simulink model "snap_hdl_pfb_v3"  (R2021a)
settings: Solver=VariableStepDiscrete  StartTime=0.0  StopTime=16384  RelTol=1e-3
undefined symbols (not defined in the file): PFB, WB_PFB
libraries: xbsIndex_r4 x451, simulink x4, xps_library x2, casper_library_misc x2
(part 1 of 6)
settings Model: Creator=wei  LastModifiedBy=wei
settings SolverCC: AlgebraicLoopSolver=TrustRegion
settings OptimizationCC: DefaultParameterBehavior=Inlined
settings DebuggingCC: SFMachineParentedDataDiag=warning
settings SFSimCC: CustomCodeUndefinedFunction=UseInterfaceOnly

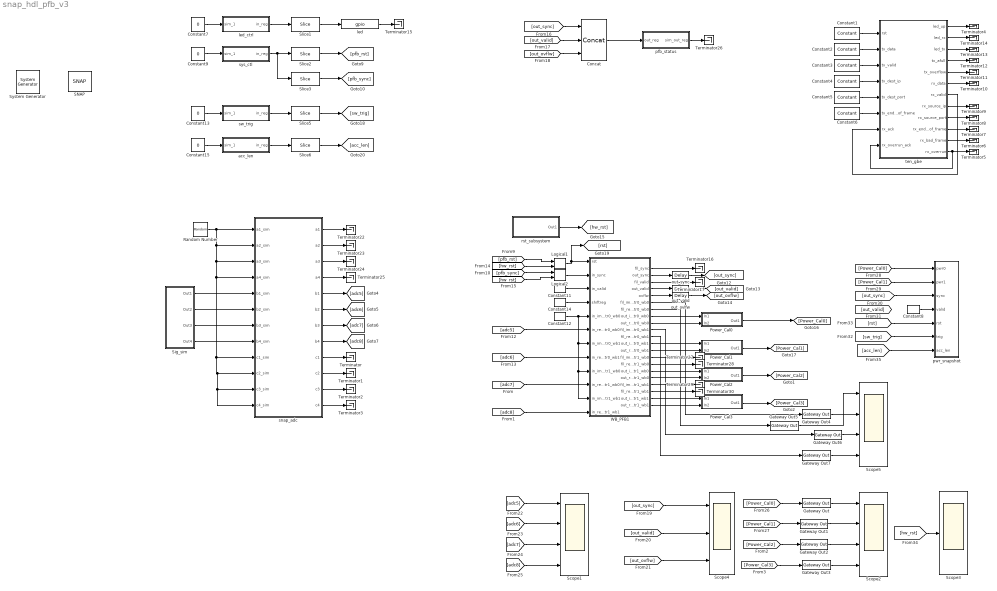
== system snap_hdl_pfb_v3 ==
  " System Generator" : xbsIndex_r4/ System Generator  Tag=genX  xilinxfamily=kintex7  part=xc7k160t  speed=-2  package=ffg676  synthesis_tool=XST  clock_wrapper=Clock Enables  directory=/data/Wei/casper_hdl/snap_hdl_tut/snap_hdl_pfb_v2/sysgen  proj_type=Vivado  Synth_file=Vivado Synthesis Defaults  Impl_file=Vivado Implementation Defaults  testbench=off  simulink_period=1  sysclk_period=4  dcm_input_clock_period=10  incr_netlist=off  trim_vbits=Everywhere in SubSystem  dbl_ovrd=According to Block Masks  core_generation=According to Block Masks  run_coregen=off  deprecated_control=off  eval_field=0  block_type=sysgen
  Concat : xbsIndex_r4/Concat  num_inputs=3  dbl_ovrd=off  block_type=concat
  Constant1 : xbsIndex_r4/Constant  const=0  gui_display_data_type=Boolean  arith_type=Boolean  n_bits=16  bin_pt=14  preci_type=Single  exp_width=8  frac_width=24  explicit_period=on  period=1  equ=P=C  opselect=C  inp2=PCIN>>17  opr=+  inp1=P  carry=CIN  dbl_ovrd=off  block_type=constant
  Constant11 : xbsIndex_r4/Constant  const=1.0  gui_display_data_type=Fixed-point  arith_type=Unsigned  n_bits=1  bin_pt=0  preci_type=Single  exp_width=8  frac_width=24  explicit_period=on  period=1  equ=P=C  opselect=C  inp2=PCIN>>17  opr=+  inp1=P  carry=CIN  dbl_ovrd=off  block_type=constant
  Constant12 : xbsIndex_r4/Constant  const=0  gui_display_data_type=Fixed-point  arith_type=Unsigned  n_bits=8  bin_pt=0  preci_type=Single  exp_width=8  frac_width=24  explicit_period=on  period=1  equ=P=C  opselect=C  inp2=PCIN>>17  opr=+  inp1=P  carry=CIN  dbl_ovrd=off  block_type=constant
  Constant{7,9,13,15} (4 alike) : Constant  Value=0  SampleTime=-1
  Constant14 : xbsIndex_r4/Constant  const=1023  gui_display_data_type=Fixed-point  arith_type=Unsigned  n_bits=10  bin_pt=0  preci_type=Single  exp_width=8  frac_width=24  explicit_period=on  period=1  equ=P=C  opselect=C  inp2=PCIN>>17  opr=+  inp1=P  carry=CIN  dbl_ovrd=off  block_type=constant
  Constant2 : xbsIndex_r4/Constant  const=0  gui_display_data_type=Fixed-point  arith_type=Unsigned  n_bits=64  bin_pt=0  preci_type=Single  exp_width=8  frac_width=24  explicit_period=on  period=1  equ=P=C  opselect=C  inp2=PCIN>>17  opr=+  inp1=P  carry=CIN  dbl_ovrd=off  block_type=constant
  Constant3 : xbsIndex_r4/Constant  const=0  gui_display_data_type=Boolean  arith_type=Boolean  n_bits=16  bin_pt=14  preci_type=Single  exp_width=8  frac_width=24  explicit_period=on  period=1  equ=P=C  opselect=C  inp2=PCIN>>17  opr=+  inp1=P  carry=CIN  dbl_ovrd=off  block_type=constant
  Constant4 : xbsIndex_r4/Constant  const=0  gui_display_data_type=Fixed-point  arith_type=Unsigned  n_bits=32  bin_pt=0  preci_type=Single  exp_width=8  frac_width=24  explicit_period=on  period=1  equ=P=C  opselect=C  inp2=PCIN>>17  opr=+  inp1=P  carry=CIN  dbl_ovrd=off  block_type=constant
  Constant5 : xbsIndex_r4/Constant  const=0  gui_display_data_type=Fixed-point  arith_type=Unsigned  n_bits=16  bin_pt=0  preci_type=Single  exp_width=8  frac_width=24  explicit_period=on  period=1  equ=P=C  opselect=C  inp2=PCIN>>17  opr=+  inp1=P  carry=CIN  dbl_ovrd=off  block_type=constant
  Constant6 : xbsIndex_r4/Constant  const=0  gui_display_data_type=Boolean  arith_type=Boolean  n_bits=32  bin_pt=0  preci_type=Single  exp_width=8  frac_width=24  explicit_period=on  period=1  equ=P=C  opselect=C  inp2=PCIN>>17  opr=+  inp1=P  carry=CIN  dbl_ovrd=off  block_type=constant
  Constant8 : xbsIndex_r4/Constant  const=1.0  gui_display_data_type=Fixed-point  arith_type=Unsigned  n_bits=1  bin_pt=0  preci_type=Single  exp_width=8  frac_width=24  explicit_period=on  period=1  equ=P=C  opselect=C  inp2=PCIN>>17  opr=+  inp1=P  carry=CIN  dbl_ovrd=off  block_type=constant
  Gateway Out{,1..7} (8 alike) : xbsIndex_r4/Gateway Out  inherit_from_input=off  hdl_port=on  rows=1  columns=1  UseAsDAC=off  DACChannel='1'  interface=None  automatic_assignment=on  address_offset=hex2dec('00')  intf_name=''  intf_description=''  timing_constraint=None  locs_specified=off  LOCs={}  io_standard={}  block_type=gatewayout
  Logical1 : xbsIndex_r4/Logical  logical_function=OR  inputs=2  en=off  latency=0  precision=Full  arith_type=Unsigned  n_bits=8  bin_pt=2  align_bp=on  dbl_ovrd=off  block_type=logical
      settings: xl_area=[0, 0, 0, 0, 0, 0, 0]
  Logical2 : xbsIndex_r4/Logical  logical_function=OR  inputs=2  en=off  latency=0  precision=Full  arith_type=Unsigned  n_bits=8  bin_pt=2  align_bp=on  dbl_ovrd=off  block_type=logical
      settings: xl_area=[0, 0, 0, 0, 0, 0, 0]
  Power_Cal0 : Subsystem
  Power_Cal1 : Subsystem
  Power_Cal2 : Subsystem
  Power_Cal3 : Subsystem
  Random Number : RandomNumber  SampleTime=0.1
  SNAP : xps_library/Platforms/SNAP  Tag=xps:xsg  hw_sys=SNAP:xc7k160t  clk_src=adc0_clk  clk_rate=250  use_microblaze=on  sample_period=1  synthesis_tool=XST
      settings: SourceProductName=CASPER XPS Blockset
  Scope1 : Scope  NumInputPorts=4
  Scope2 : Scope  NumInputPorts=4
  Scope3 : Scope
  Scope4 : Scope  NumInputPorts=3
  Scope5 : Scope  NumInputPorts=4
  Sig_sim : Subsystem
  Slice1 : xbsIndex_r4/Slice  nbits=1  boolean_output=on  mode=Lower Bit Location + Width  bit1=0  base1=MSB of Input  bit0=0  base0=LSB of Input  dbl_ovrd=off  block_type=slice
  Slice2 : xbsIndex_r4/Slice  nbits=1  boolean_output=on  mode=Lower Bit Location + Width  bit1=0  base1=MSB of Input  bit0=0  base0=LSB of Input  dbl_ovrd=off  block_type=slice
  Slice3 : xbsIndex_r4/Slice  nbits=1  boolean_output=on  mode=Lower Bit Location + Width  bit1=0  base1=MSB of Input  bit0=1  base0=LSB of Input  dbl_ovrd=off  block_type=slice
  Slice5 : xbsIndex_r4/Slice  nbits=10  boolean_output=on  mode=Lower Bit Location + Width  bit1=0  base1=MSB of Input  bit0=0  base0=LSB of Input  dbl_ovrd=off  block_type=slice
  Slice6 : xbsIndex_r4/Slice  nbits=24  boolean_output=off  mode=Lower Bit Location + Width  bit1=0  base1=MSB of Input  bit0=0  base0=LSB of Input  dbl_ovrd=off  block_type=slice
  Terminator{,1..17,22..30} (27 alike) : Terminator
  WB_PFB1 : Subsystem  AncestorBlock=PFB/WB_PFB  mask(Wideband Polyphase Filterbank Block){use_separate=off, use_fft_shift=off, use_reorder=on, alt_output=off, wb_factor=2, nof_points=10, nof_taps=4, nof_wb_streams=2, nof_chan=0, xtra_dat_sigs=off, big_endian_wb_in=off, use_prefilter=on, dont_flip_channels=on, out_gain_w=0, win="hanning", fwidth=1.0, backoff_w=0, fil_in_dat_w=8, fil_out_dat_w=14, fil_coef_dat_w=10, twid_dat_w=18, fft_stage_dat_w=20, fft_out_dat_w=20, fft_guard_enable=off, fft_guard_w=2, fft_ovflw_behav="WRAP", fft_use_round=1, pipe_reo_in_place=off, use_dsp="YES", use_variant="4DSP", fft_ram_primitive="block", max_addr_w=8, fil_ram_primitive="block", vendor_technology=Xilinx}
      mask prompts: use_separate "Separate re/im outputs"; use_fft_shift "Reorder frequencies"; use_reorder "Bit reverse output"; alt_output "Alter output data stream"; wb_factor "Wideband factor"; nof_points "Number of points (2^nof_pts)"; nof_taps "Number of taps"; nof_wb_streams "Number of wideband streams"; nof_chan "Number of channels (2^nof_chan)"; xtra_dat_sigs "Extra control signals"; big_endian_wb_in "Big endian input data"; use_prefilter "Enable prefilter"; dont_flip_channels "Don't flip channels"; out_gain_w "Output gain width"; win "Window function"; backoff_w "Filter backoff width"; fil_in_dat_w "Prefilter input data width"; fil_out_dat_w "Prefilter output data width"; fil_coef_dat_w "Prefilter coefficient data width"; twid_dat_w "FFT twiddle data width"; fft_stage_dat_w "FFT stage data width"; fft_out_dat_w "FFT output data width"; fft_guard_enable "Guard FFT input data"; fft_guard_w "FFT guard data width"; fft_ovflw_behav "FFT overflow behaviour"; fft_use_round "FFT rounding mode: 0-Truncate, 1-Round Even, 2-Round Infinite"; pipe_reo_in_place "Use single pipelined FFT reorder buffer"; use_dsp "Use DSP for Cmults"; use_variant "Cmult options"; fft_ram_primitive "FFT Ram Primitive"; max_addr_w "Twiddle Max Address Width"; fil_ram_primitive "Prefilter Ram Primitive"; vendor_technology "Vendor technology"
      mask help: The Wideband Poly Phase FilterBank can process a datastream that is partly applied in serial and partly applied in parallel. It consists of a Poly Phase Filter (PPF) and a Fast Fourier Transform (FFT). It distinguishes from a single FFT by the PPF, that acts as a window function to produce a flat response across the channel, and excellent suppression of out-of-band signals.
      mask init:
      | Simulink.Block.eval([gcb, '/wb_pfb']);
      |  
      | wb_pfb_subsys2bb_knit();
      mask Help: https://casper-dspdevel.readthedocs.io/en/latest/wideband_pfb.html
      mask Callback use_separate:
      | enab = get_param(gcb,'use_separate');
      | 
      | % Set the 'MaskVisibilities' property for each parameters
      | if strcmp(enab,'on')
      |     set_param(gcb,'use_reorder','on');
      |     set_param(gcb,'use_fft_shift','off');
      |     set_param(gcb,'MaskEnables',{'on','off','off','on','on','on','on','on','on','on','on','on','on','on','on','on','on','on','on','on','on','on','on','on','on','on','on','on','on','on','on','on','on','on'});
      | else
      |     set_param(gcb,'MaskEnables',{'on','on','on','on','on','on','on','on','on','on','on','on','on','on','on','on','on','on','on','on','on','on','on','on','on','on','on','on','on','on','on','on','on','on'});
      | end
      mask Callback use_fft_shift:
      | enab = get_param(gcb,'use_fft_shift');
      | 
      | % Set the 'MaskVisibilities' property for each parameters
      | if strcmp(enab,'on')
      |     set_param(gcb,'use_reorder','on');
      |     set_param(gcb,'MaskEnables',{'on','on','off','on','on','on','on','on','on','on','on','on','on','on','on','on','on','on','on','on','on','on','on','on','on','on','on','on','on','on','on','on','on','on'});
      | else
      |     set_param(gcb,'MaskEnables',{'on','on','on','on','on','on','on','on','on','on','on','on','on','on','on','on','on','on','on','on','on','on','on','on','on','on','on','on','on','on','on','on','on','on'});
      | end
      mask TypeOptions win: "hanning" | "hamming" | "blackman"
      mask Callback fft_guard_enable:
      | enab = get_param(gcb,'fft_guard_enable');
      | 
      | % Set the 'MaskVisibilities' property for each parameters
      | if strcmp(enab,'on')
      |     set_param(gcb,'MaskVisibilities',{'on','on','on','on','on','on','on','on','on','on','on','on','on','on','on','on','on','on','on','on','on','on','on','on','on','on','on','on','on','on','on','on','on','on'});
      | else
      |     set_param(gcb,'MaskVisibilities',{'on','on','on','on','on','on','on','on','on','on','on','on','on','on','on','on','on','on','on','on','on','on','on','on','off','on','on','on','on','on','on','on','on','on'});
      | end
      mask TypeOptions fft_ovflw_behav: "SATURATE" | "WRAP"
      mask TypeOptions fft_use_round: 0 | 1 | 2
      mask TypeOptions use_dsp: "YES" | "NO"
      mask TypeOptions use_variant: "4DSP" | "3DSP"
      mask TypeOptions fft_ram_primitive: "block" | "distributed" | "ultra" | "auto"
      mask TypeOptions fil_ram_primitive: "block" | "distributed" | "ultra" | "auto"
      mask TypeOptions vendor_technology: Xilinx | UniBoard
      mask DialogControl DescTextVar Prompt: The wpfb unit is a Wideband Poly Phase FilterBank which can process a datastream that is partly applied in serial and partly applied in parallel. It consists of a Poly Phase Filter (PPF) and a Fast Fourier Transform (FFT). The wpfb distinguishes from a single FFT by the PPF that functions as a window function in order to produce a flat response across the channel, but also provides excellent suppression of out-of-band signals. https://casper-dspdevel.readthedocs.io/en/latest/wideband_pfb.html
      mask DialogControl pfb_params Prompt: PFB Parameters
      mask DialogControl pfb Prompt: PFB
      mask DialogControl filter Prompt: FILTER
      mask DialogControl fft Prompt: FFT
      mask DialogControl synth Prompt: SYNTH/IMP
  acc_len : Subsystem  Tag=xps:sw_reg  AncestorBlock=xps_library/Memory/software_register  mask(swreg){io_dir=From Processor, io_delay=0, init_val=0, sample_period=1, names=reg, bitwidths=32, bin_pts=0, arith_types=0, sim_port=on, show_format=on}
      mask prompts: io_dir "I/O direction"; io_delay "I/O delay"; init_val "Initial Value"; sample_period "Sample period"; names "Bitfield names [msb...lsb]"; bitwidths "Bitfield widths"; bin_pts "Bitfield binary pts"; arith_types "Bitfield types, ufix=0, fix=1, bool=2"; sim_port "Provide sim input/output?"; show_format "Print format string?"
      mask help: A 32-bit software-accessible register. Can be divided into bitfields of varying widths and types using the fields in the block mask.
      mask init:
      | swreg_init(gcb)
      settings: AttributesFormatString=1input:uf32.0 = 32 bits
      mask TypeOptions io_dir: To Processor | From Processor
      mask Callback io_dir:
      | mask_enables = get_param(gcb, 'MaskEnables');
      | mask_names = get_param(gcb, 'MaskNames');
      | if strcmp(get_param(gcb, 'io_dir'), 'To Processor'),
      |     mask_enables{ismember(mask_names, 'sample_period')} = 'off';
      | else
      |     mask_enables{ismember(mask_names, 'sample_period')} = 'on';
      | end
      | set_param(gcb, 'MaskEnables', mask_enables);
      mask DialogControl ParameterTabVar0 Prompt: Setup
  led : xps_library/IO/gpio  Tag=xps:gpio  io_group_params_forwarded=on  io_group=ROACH:led  io_group_real=led  io_group_custom=0  io_dir=out  arith_type=Boolean  bitwidth=1  bin_pt=0  bit_index=0  sample_period=1  use_single_ended=off  use_ddr=off  reg_iob=on  reg_clk_phase=0  termination=None  use_iodelay=off
      settings: SourceProductName=CASPER XPS Blockset
  led_ctrl : Subsystem  Tag=xps:sw_reg  AncestorBlock=xps_library/Memory/software_register  mask(swreg){io_dir=From Processor, io_delay=0, init_val=0, sample_period=1, names=reg, bitwidths=32, bin_pts=0, arith_types=0, sim_port=on, show_format=on}
      mask prompts: io_dir "I/O direction"; io_delay "I/O delay"; init_val "Initial Value"; sample_period "Sample period"; names "Bitfield names [msb...lsb]"; bitwidths "Bitfield widths"; bin_pts "Bitfield binary pts"; arith_types "Bitfield types, ufix=0, fix=1, bool=2"; sim_port "Provide sim input/output?"; show_format "Print format string?"
      mask help: A 32-bit software-accessible register. Can be divided into bitfields of varying widths and types using the fields in the block mask.
      mask init:
      | swreg_init(gcb)
      settings: AttributesFormatString=1input:uf32.0 = 32 bits
      mask TypeOptions io_dir: To Processor | From Processor
      mask Callback io_dir:
      | mask_enables = get_param(gcb, 'MaskEnables');
      | mask_names = get_param(gcb, 'MaskNames');
      | if strcmp(get_param(gcb, 'io_dir'), 'To Processor'),
      |     mask_enables{ismember(mask_names, 'sample_period')} = 'off';
      | else
      |     mask_enables{ismember(mask_names, 'sample_period')} = 'on';
      | end
      | set_param(gcb, 'MaskEnables', mask_enables);
      mask DialogControl ParameterTabVar0 Prompt: Setup
  out_ovlfw : xbsIndex_r4/Delay  rst=off  infoeditControl=Selection of Reset will increase slice count due to use of real FFs and instead of SRLs  en=off  latency=5  reg_retiming=off  dbl_ovrd=off  block_type=delay
  out_sync : xbsIndex_r4/Delay  rst=off  infoeditControl=Selection of Reset will increase slice count due to use of real FFs and instead of SRLs  en=off  latency=5  reg_retiming=off  dbl_ovrd=off  block_type=delay
  out_valid : xbsIndex_r4/Delay  rst=off  infoeditControl=Selection of Reset will increase slice count due to use of real FFs and instead of SRLs  en=off  latency=5  reg_retiming=off  dbl_ovrd=off  block_type=delay
  pfb_status : Subsystem  Tag=xps:sw_reg  AncestorBlock=xps_library/Memory/software_register  mask(swreg){io_dir=To Processor, io_delay=0, init_val=0, sample_period=1, names=reg, bitwidths=12, bin_pts=0, arith_types=0, sim_port=on, show_format=off}
      mask prompts: io_dir "I/O direction"; io_delay "I/O delay"; init_val "Initial Value"; sample_period "Sample period"; names "Bitfield names [msb...lsb]"; bitwidths "Bitfield widths"; bin_pts "Bitfield binary pts"; arith_types "Bitfield types, ufix=0, fix=1, bool=2"; sim_port "Provide sim input/output?"; show_format "Print format string?"
      mask help: A 32-bit software-accessible register. Can be divided into bitfields of varying widths and types using the fields in the block mask.
      mask init:
      | swreg_init(gcb)
      settings: AttributesFormatString=1output
      mask TypeOptions io_dir: To Processor | From Processor
      mask Callback io_dir:
      | mask_enables = get_param(gcb, 'MaskEnables');
      | mask_names = get_param(gcb, 'MaskNames');
      | if strcmp(get_param(gcb, 'io_dir'), 'To Processor'),
      |     mask_enables{ismember(mask_names, 'sample_period')} = 'off';
      | else
      |     mask_enables{ismember(mask_names, 'sample_period')} = 'on';
      | end
      | set_param(gcb, 'MaskEnables', mask_enables);
      mask DialogControl ParameterTabVar0 Prompt: Setup
  pwr_snapshot : Subsystem
  rst_subsystem : Subsystem
  snap_adc : Subsystem  Tag=xps:snap_adc  AncestorBlock=xps_library/ADCs/snap_adc  mask(adc_snap){sample_rate=500, snap_inputs=6, adc_resolution=8}
      mask prompts: sample_rate "Sample rate (MHz)"; snap_inputs "Number of inputs per snap"; adc_resolution "Resolution of ADC (number of bit)"
      mask help: Interface to the 3 adc chips on the SNAP board. Please see Help for instructions on parameter settings
      mask init:
      | adc_snap_init(gcb);
      mask Help:
      | This is the CASPER "yellow block" for the ADCs on the SNAP board.
      | Each ADC chip accepts four inputs.
      | 
      | Maximum sample rate f (Mega samples per second)
      | 
      | Number of inputs         3                6                12
      | Resolution 8 bits          f=1000      f=500         f=250
      | Resolution 12 bits        f=640        f=320         f=160
      | 
      | Resolution 12 bits is available when SNAP board is upgraded with HMCAD1520 ADC chips
      mask TypeOptions snap_inputs: 3 | 6 | 12
      mask TypeOptions adc_resolution: 8 | 12
  sw_trig : Subsystem  Tag=xps:sw_reg  AncestorBlock=xps_library/Memory/software_register  mask(swreg){io_dir=From Processor, io_delay=0, init_val=0, sample_period=1, names=reg, bitwidths=32, bin_pts=0, arith_types=0, sim_port=on, show_format=on}
      mask prompts: io_dir "I/O direction"; io_delay "I/O delay"; init_val "Initial Value"; sample_period "Sample period"; names "Bitfield names [msb...lsb]"; bitwidths "Bitfield widths"; bin_pts "Bitfield binary pts"; arith_types "Bitfield types, ufix=0, fix=1, bool=2"; sim_port "Provide sim input/output?"; show_format "Print format string?"
      mask help: A 32-bit software-accessible register. Can be divided into bitfields of varying widths and types using the fields in the block mask.
      mask init:
      | swreg_init(gcb)
      settings: AttributesFormatString=1input:uf32.0 = 32 bits
      mask TypeOptions io_dir: To Processor | From Processor
      mask Callback io_dir:
      | mask_enables = get_param(gcb, 'MaskEnables');
      | mask_names = get_param(gcb, 'MaskNames');
      | if strcmp(get_param(gcb, 'io_dir'), 'To Processor'),
      |     mask_enables{ismember(mask_names, 'sample_period')} = 'off';
      | else
      |     mask_enables{ismember(mask_names, 'sample_period')} = 'on';
      | end
      | set_param(gcb, 'MaskEnables', mask_enables);
      mask DialogControl ParameterTabVar0 Prompt: Setup
  sys_ctl : Subsystem  Tag=xps:sw_reg  AncestorBlock=xps_library/Memory/software_register  mask(swreg){io_dir=From Processor, io_delay=0, init_val=0, sample_period=1, names=reg, bitwidths=32, bin_pts=0, arith_types=0, sim_port=on, show_format=on}
      mask prompts: io_dir "I/O direction"; io_delay "I/O delay"; init_val "Initial Value"; sample_period "Sample period"; names "Bitfield names [msb...lsb]"; bitwidths "Bitfield widths"; bin_pts "Bitfield binary pts"; arith_types "Bitfield types, ufix=0, fix=1, bool=2"; sim_port "Provide sim input/output?"; show_format "Print format string?"
      mask help: A 32-bit software-accessible register. Can be divided into bitfields of varying widths and types using the fields in the block mask.
      mask init:
      | swreg_init(gcb)
      settings: AttributesFormatString=1input:uf32.0 = 32 bits
      mask TypeOptions io_dir: To Processor | From Processor
      mask Callback io_dir:
      | mask_enables = get_param(gcb, 'MaskEnables');
      | mask_names = get_param(gcb, 'MaskNames');
      | if strcmp(get_param(gcb, 'io_dir'), 'To Processor'),
      |     mask_enables{ismember(mask_names, 'sample_period')} = 'off';
      | else
      |     mask_enables{ismember(mask_names, 'sample_period')} = 'on';
      | end
      | set_param(gcb, 'MaskEnables', mask_enables);
      mask DialogControl ParameterTabVar0 Prompt: Setup
  ten_gbe : Subsystem  Tag=xps:ten_gbe  AncestorBlock=xps_library/IO/ten_gbe  mask(ten_gbe){flavour=sfp+, slot=0, port_r1=1, port_r2_cx4=0, port_r2_sfpp=0, rx_dist_ram=off, large_frames=on, show_param=on, pre_emph_r2=1.07, pre_emph=3, post_emph_r2=0.18, rxeqmix_r2=7, swing_r2=940, swing=800, fab_en=off, fab_mac=hex2dec('123456780000'), fab_ip=192*(2^24) + 168*(2^16) + 5*(2^8) + 20*(2^0), fab_udp=10000, fab_gate=1, cpu_rx_en=on, cpu_tx_en=on, ttl=hex2dec('FF'), promisc_mode=off, debug_ctr_width=16, txctr=off, txerrctr=off, txerrctr_len=100, txofctr=off, txfullctr=off, txvldctr=off, txsnaplen=0 - no snap, rxctr=off, rxerrctr=off, rxerrctr_len=100, rxofctr=off, rxbadctr=off, rxvldctr=off, rxeofctr=off, rxsnaplen=0 - no snap}
      mask prompts: flavour "Mezzanine card flavour"; slot "Card slot"; port_r1 "Port"; port_r2_cx4 "Port"; port_r2_sfpp "Port"; rx_dist_ram "Shallow RX Fifo (Beware overruns!)"; large_frames "Enable Large TX Frames (8k+512)"; show_param "---------------------- Show Implementation Parameters -----------------------------------------------------------------------------------"; pre_emph_r2 "Pre-emphasis (dB)"; pre_emph "Pre-emphasis"; post_emph_r2 "Post-emphasis (dB)"; rxeqmix_r2 "Receive equalisation"; swing_r2 "Driver Swing Control (mVppd)"; swing "Differential swing"; fab_en "Enable fabric on startup"; fab_mac "Fabric MAC Address"; fab_ip "Fabric IP Address"; fab_udp "Fabric UDP Port"; fab_gate "Fabric Gateway"; cpu_rx_en "Enable CPU RX"; cpu_tx_en "Enable CPU TX"; promisc_mode "Promiscuous mode"; debug_ctr_width "Debug counter width"; txctr "TX - core_txctr"; txerrctr "TX packet length error - core_txerrctr"; txerrctr_len "-- expected TX packet length"; txofctr "TX overflow - core_txofctr"; txfullctr "TX full - core_txfullctr"; txvldctr "TX valid cycle - core_txvldctr"; txsnaplen "TX snapshot length"; rxctr "RX - core_rxctr"; rxerrctr "RX packet length error - core_rxerrctr"; rxerrctr_len "-- expected RX packet length"; rxofctr "RX overflow - core_rxofctr"; rxbadctr "RX bad - core_rxbadctr"; rxvldctr "RX valid cycle - core_rxvldctr"; rxeofctr "RX eof - core_rxeofctr"; rxsnaplen "RX snapshot length"
      mask help: This block sends and receives UDP frames (packets). It accepts a 64 bit wide data stream with user-determined frame breaks. The data stream is wrapped in a UDP frame for transmission. Incoming UDP packets are unwrapped and the data presented as a 64 bit wide stream.
      mask init:
      | temp = eval(get_param(gcb, 'debug_ctr_width'));
      | if temp <= 0,
      |     error('Debug counters cannot be ltoet zero.');
      | end
      | tengbe_mask(gcb)
      mask TypeOptions flavour: sfp+ | cx4
      mask Callback flavour: tengbe_callback
      mask TypeOptions slot: 0 | 1
      mask TypeOptions port_r1: 0 | 1 | 2 | 3
      mask TypeOptions port_r2_cx4: 0 | 1 | 2
      mask TypeOptions port_r2_sfpp: 0 | 1 | 2 | 3
      mask Callback show_param: tengbe_callback
      mask TypeOptions pre_emph_r2: 0.15 | 0.3 | 0.45 | 0.61 | 0.74 | 0.91 | 1.07 | 1.25 | 1.36 | 1.55 | 1.74 | 1.94 | 2.11 | 2.32 | 2.54 | 2.77
      mask TypeOptions pre_emph: 0 | 1 | 2 | 3
      mask TypeOptions post_emph_r2: 0.18 | 0.19 | 0.2 | 0.39 | 0.63 | 0.82 | 1.07 | 1.32 | 1.6 | 1.65 | 1.94 | 2.21 | 2.52 | 2.76 | 3.08 | 3.41 | 3.77 | 3.97 | 4.36 | 4.73 | 5.16 | 5.47 | 5.93 | 6.38 | 6.89
      mask TypeOptions rxeqmix_r2: 0 | 1 | 2 | 3 | 4 | 5 | 6 | 7
      mask TypeOptions swing_r2: 110 | 210 | 310 | 400 | 480 | 570 | 660 | 740 | 810 | 880 | 940 | 990 | 1040 | 1080 | 1110 | 1130
      mask TypeOptions swing: 400 | 500 | 600 | 700 | 800
      mask Callback txerrctr:
      | blk = gcb;
      | mask_visibilities = get_param(blk, 'MaskVisibilities');
      | mask_names = get_param(blk, 'MaskNames');
      | if strcmp(get_param(blk, 'txerrctr'), 'on')
      |     mask_visibilities{ismember(mask_names, 'txerrctr_len')} = 'on';
      | else
      |     mask_visibilities{ismember(mask_names, 'txerrctr_len')} = 'off';
      | end
      | set_param(blk, 'MaskVisibilities', mask_visibilities);
      mask TypeOptions txsnaplen: 0 - no snap | 256 | 512 | 1024 | 2048 | 4096 | 8192 | 16384
      mask Callback rxerrctr:
      | blk = gcb;
      | mask_visibilities = get_param(blk, 'MaskVisibilities');
      | mask_names = get_param(blk, 'MaskNames');
      | if strcmp(get_param(blk, 'rxerrctr'), 'on')
      |     mask_visibilities{ismember(mask_names, 'rxerrctr_len')} = 'on';
      | else
      |     mask_visibilities{ismember(mask_names, 'rxerrctr_len')} = 'off';
      | end
      | set_param(blk, 'MaskVisibilities', mask_visibilities);
      mask TypeOptions rxsnaplen: 0 - no snap | 256 | 512 | 1024 | 2048 | 4096 | 8192 | 16384
      mask DialogControl ParameterTabVar0 Prompt: Core
      mask DialogControl ParameterTabVar01 Prompt: Debug counters
  wires:
  snap_adc/1(a1) -> Terminator22/1
  snap_adc/4(a4) -> Terminator25/1
  snap_adc/3(a3) -> Terminator24/1
  snap_adc/2(a2) -> Terminator23/1
  snap_adc/9(c1) -> Terminator/1
  snap_adc/11(c3) -> Terminator2/1
  snap_adc/10(c2) -> Terminator1/1
  snap_adc/12(c4) -> Terminator3/1
  Random Number/1 -> snap_adc/2(a2_sim), snap_adc/12(c4_sim), snap_adc/11(c3_sim), snap_adc/10(c2_sim), snap_adc/9(c1_sim), snap_adc/4(a4_sim), snap_adc/3(a3_sim), snap_adc/1(a1_sim)
  ten_gbe/1(led_up) -> Terminator4/1
  Constant1/1 -> ten_gbe/1(rst)
  Constant2/1 -> ten_gbe/2(tx_data)
  Constant3/1 -> ten_gbe/3(tx_valid)
  Constant4/1 -> ten_gbe/4(tx_dest_ip)
  Constant5/1 -> ten_gbe/5(tx_dest_port)
  Constant6/1 -> ten_gbe/6(tx_end_of_frame)
  ten_gbe/7(rx_valid) -> ten_gbe/7(rx_ack)
  ten_gbe/12(rx_overrun) -> Terminator5/1, ten_gbe/8(rx_overrun_ack)
  ten_gbe/11(rx_bad_frame) -> Terminator6/1
  ten_gbe/10(rx_end_of_frame) -> Terminator7/1
  ten_gbe/9(rx_source_port) -> Terminator8/1
  ten_gbe/8(rx_source_ip) -> Terminator9/1
  ten_gbe/6(rx_data) -> Terminator10/1
  ten_gbe/5(tx_overflow) -> Terminator11/1
  ten_gbe/4(tx_afull) -> Terminator12/1
  ten_gbe/3(led_tx) -> Terminator13/1
  ten_gbe/2(led_rx) -> Terminator14/1
  Constant7/1 -> led_ctrl/1(sim_1)
  led/1 -> Terminator15/1
  Slice1/1 -> led/1
  led_ctrl/1(in_reg) -> Slice1/1
  sys_ctl/1(in_reg) -> Slice3/1, Slice2/1
  Constant9/1 -> sys_ctl/1(sim_1)
  Slice2/1 -> [pfb_rst]
  Slice3/1 -> [pfb_sync]
  Constant11/1 -> WB_PFB1/3(in_valid)
  WB_PFB1/1(fil_sync) -> Terminator16/1
  WB_PFB1/3(fil_valid) -> Terminator17/1
  WB_PFB1/2(out_sync) -> out_sync/1
  WB_PFB1/4(out_valid) -> out_valid/1
  WB_PFB1/5(ovflw) -> out_ovlfw/1
  [out_sync] -> Concat/1
  [out_valid] -> Concat/2
  [out_ovflw] -> Concat/3
  Concat/1 -> pfb_status/1(out_reg)
  pfb_status/1(sim_out_reg) -> Terminator26/1
  [adc5] -> Scope1/1
  [adc6] -> Scope1/2
  [adc7] -> Scope1/3
  [adc8] -> Scope1/4
  Constant14/1 -> WB_PFB1/4(shiftreg)
  snap_adc/5(b1) -> [adc5]
  snap_adc/6(b2) -> [adc6]
  snap_adc/7(b3) -> [adc7]
  snap_adc/8(b4) -> [adc8]
  Power_Cal0/1(Out1) -> [Power_Cal0]
  Power_Cal1/1(Out1) -> [Power_Cal1]
  [out_ovflw] -> Scope4/3
  [out_valid] -> Scope4/2
  [out_sync] -> Scope4/1
  Logical2/1 -> WB_PFB1/2(in_sync)
  WB_PFB1/6(fil_im_str0_wb0) -> Gateway Out4/1
  Constant12/1 -> WB_PFB1/9(in_im_str1_wb0), WB_PFB1/11(in_im_str1_wb1), WB_PFB1/7(in_im_str0_wb1), WB_PFB1/5(in_im_str0_wb0)
  [pfb_rst] -> Logical1/1
  [hw_rst] -> Logical1/2
  Logical1/1 -> WB_PFB1/1(rst), [rst]
  [hw_rst] -> Logical2/2
  [pfb_sync] -> Logical2/1
  out_sync/1 -> [out_sync]
  out_valid/1 -> [out_valid]
  [Power_Cal0] -> pwr_snapshot/1(pwr0)
  [Power_Cal1] -> pwr_snapshot/2(pwr1)
  [out_sync] -> pwr_snapshot/3(sync)
  Sig_sim/4(Out4) -> snap_adc/8(b4_sim)
  Sig_sim/1(Out1) -> snap_adc/5(b1_sim)
  Sig_sim/2(Out2) -> snap_adc/6(b2_sim)
  Sig_sim/3(Out3) -> snap_adc/7(b3_sim)
  out_ovlfw/1 -> [out_ovflw]
  sw_trig/1(in_reg) -> Slice5/1
  Constant13/1 -> sw_trig/1(sim_1)
  Slice5/1 -> [sw_trig]
  [sw_trig] -> pwr_snapshot/6(trig)
  [rst] -> pwr_snapshot/5(rst)
  [hw_rst] -> Scope3/1
  rst_subsystem/1(Out1) -> [hw_rst]
  Constant15/1 -> acc_len/1(sim_1)
  acc_len/1(in_reg) -> Slice6/1
  [acc_len] -> pwr_snapshot/7(acc_len)
  Slice6/1 -> [acc_len]
  [adc5] -> WB_PFB1/6(in_re_str0_wb0)
  [adc6] -> WB_PFB1/8(in_re_str0_wb1)
  WB_PFB1/7(fil_re_str0_wb0) -> Gateway Out5/1
  WB_PFB1/8(out_im_str0_wb0) -> Power_Cal0/1(In1)
  WB_PFB1/9(out_re_str0_wb0) -> Power_Cal0/2(In2)
  WB_PFB1/11(fil_re_str0_wb1) -> Gateway Out7/1
  WB_PFB1/12(out_im_str0_wb1) -> Power_Cal1/1(In1)
  WB_PFB1/13(out_re_str0_wb1) -> Power_Cal1/2(In2)
  [adc7] -> WB_PFB1/10(in_re_str1_wb0)
  [adc8] -> WB_PFB1/12(in_re_str1_wb1)
  WB_PFB1/14(fil_im_str1_wb0) -> Terminator27/1
  WB_PFB1/15(fil_re_str1_wb0) -> Terminator28/1
  WB_PFB1/16(out_im_str1_wb0) -> Power_Cal2/1(In1)
  WB_PFB1/17(out_re_str1_wb0) -> Power_Cal2/2(In2)
  WB_PFB1/20(out_im_str1_wb1) -> Power_Cal3/1(In1)
  WB_PFB1/21(out_re_str1_wb1) -> Power_Cal3/2(In2)
  WB_PFB1/18(fil_im_str1_wb1) -> Terminator29/1
  WB_PFB1/19(fil_re_str1_wb1) -> Terminator30/1
  Power_Cal2/1(Out1) -> [Power_Cal2]
  Power_Cal3/1(Out1) -> [Power_Cal3]
  [Power_Cal0] -> Gateway Out/1
  [Power_Cal1] -> Gateway Out1/1
  [Power_Cal3] -> Gateway Out3/1
  [Power_Cal2] -> Gateway Out2/1
  Gateway Out1/1 -> Scope2/2
  Gateway Out/1 -> Scope2/1
  Gateway Out2/1 -> Scope2/3
  Gateway Out3/1 -> Scope2/4
  Gateway Out4/1 -> Scope5/2
  Gateway Out5/1 -> Scope5/1
  Gateway Out6/1 -> Scope5/3
  Gateway Out7/1 -> Scope5/4
  WB_PFB1/10(fil_im_str0_wb1) -> Gateway Out6/1
  Constant8/1 -> pwr_snapshot/4(valid)

== system snap_hdl_pfb_v3/Power_Cal0 ==
  In1 : Inport
  In2 : Inport  Port=2
  AddSub : xbsIndex_r4/AddSub  mode=Addition  use_carryin=off  use_carryout=off  en=off  latency=2  precision=User Defined  arith_type=Unsigned  n_bits=40  bin_pt=0  quantization=Truncate  overflow=Wrap  use_behavioral_HDL=off  hw_selection=Fabric  pipelined=off  dbl_ovrd=off  block_type=addsub
  Mult : xbsIndex_r4/Mult  precision=Full  arith_type=Unsigned  n_bits=36  bin_pt=0  quantization=Truncate  overflow=Wrap  en=off  latency=3  use_behavioral_HDL=off  opt=Speed  use_embedded=on  optimum_pipeline=off  pipeline=on  dbl_ovrd=off  use_rpm=on  placement_style=Triangular  block_type=mult
  Mult1 : xbsIndex_r4/Mult  precision=Full  arith_type=Unsigned  n_bits=36  bin_pt=0  quantization=Truncate  overflow=Wrap  en=off  latency=3  use_behavioral_HDL=off  opt=Speed  use_embedded=on  optimum_pipeline=off  pipeline=on  dbl_ovrd=off  use_rpm=on  placement_style=Triangular  block_type=mult
  Reinterpret : xbsIndex_r4/Reinterpret  force_arith_type=on  arith_type="Signed  (2's comp)"  force_bin_pt=on  bin_pt=0  block_type=reinterpret
  Reinterpret1 : xbsIndex_r4/Reinterpret  force_arith_type=on  arith_type="Signed  (2's comp)"  force_bin_pt=on  bin_pt=0  block_type=reinterpret
  Slice_im : xbsIndex_r4/Slice  nbits=20  boolean_output=off  mode=Upper Bit Location + Width  bit1=0  base1=MSB of Input  bit0=0  base0=LSB of Input  dbl_ovrd=off  block_type=slice
  Slice_re : xbsIndex_r4/Slice  nbits=20  boolean_output=off  mode=Upper Bit Location + Width  bit1=0  base1=MSB of Input  bit0=0  base0=LSB of Input  dbl_ovrd=off  block_type=slice
  Out1 : Outport
  wires:
  In2/1 -> Slice_im/1
  In1/1 -> Slice_re/1
  Reinterpret/1 -> Mult/1, Mult/2
  Reinterpret1/1 -> Mult1/2, Mult1/1
  Mult/1 -> AddSub/1
  Mult1/1 -> AddSub/2
  AddSub/1 -> Out1/1
  Slice_re/1 -> Reinterpret/1
  Slice_im/1 -> Reinterpret1/1

== system snap_hdl_pfb_v3/Power_Cal1 ==
  In1 : Inport
  In2 : Inport  Port=2
  AddSub : xbsIndex_r4/AddSub  mode=Addition  use_carryin=off  use_carryout=off  en=off  latency=2  precision=User Defined  arith_type=Unsigned  n_bits=40  bin_pt=0  quantization=Truncate  overflow=Wrap  use_behavioral_HDL=off  hw_selection=Fabric  pipelined=off  dbl_ovrd=off  block_type=addsub
  Mult : xbsIndex_r4/Mult  precision=Full  arith_type=Unsigned  n_bits=36  bin_pt=0  quantization=Truncate  overflow=Wrap  en=off  latency=3  use_behavioral_HDL=off  opt=Speed  use_embedded=on  optimum_pipeline=off  pipeline=on  dbl_ovrd=off  use_rpm=on  placement_style=Triangular  block_type=mult
  Mult1 : xbsIndex_r4/Mult  precision=Full  arith_type=Unsigned  n_bits=36  bin_pt=0  quantization=Truncate  overflow=Wrap  en=off  latency=3  use_behavioral_HDL=off  opt=Speed  use_embedded=on  optimum_pipeline=off  pipeline=on  dbl_ovrd=off  use_rpm=on  placement_style=Triangular  block_type=mult
  Reinterpret : xbsIndex_r4/Reinterpret  force_arith_type=on  arith_type="Signed  (2's comp)"  force_bin_pt=on  bin_pt=0  block_type=reinterpret
  Reinterpret1 : xbsIndex_r4/Reinterpret  force_arith_type=on  arith_type="Signed  (2's comp)"  force_bin_pt=on  bin_pt=0  block_type=reinterpret
  Slice_im : xbsIndex_r4/Slice  nbits=20  boolean_output=off  mode=Upper Bit Location + Width  bit1=0  base1=MSB of Input  bit0=0  base0=LSB of Input  dbl_ovrd=off  block_type=slice
  Slice_re : xbsIndex_r4/Slice  nbits=20  boolean_output=off  mode=Upper Bit Location + Width  bit1=0  base1=MSB of Input  bit0=0  base0=LSB of Input  dbl_ovrd=off  block_type=slice
  Out1 : Outport
  wires:
  In2/1 -> Slice_im/1
  In1/1 -> Slice_re/1
  Reinterpret/1 -> Mult/1, Mult/2
  Reinterpret1/1 -> Mult1/2, Mult1/1
  Mult/1 -> AddSub/1
  Mult1/1 -> AddSub/2
  AddSub/1 -> Out1/1
  Slice_re/1 -> Reinterpret/1
  Slice_im/1 -> Reinterpret1/1

== system snap_hdl_pfb_v3/Power_Cal2 ==
  In1 : Inport
  In2 : Inport  Port=2
  AddSub : xbsIndex_r4/AddSub  mode=Addition  use_carryin=off  use_carryout=off  en=off  latency=2  precision=User Defined  arith_type=Unsigned  n_bits=40  bin_pt=0  quantization=Truncate  overflow=Wrap  use_behavioral_HDL=off  hw_selection=Fabric  pipelined=off  dbl_ovrd=off  block_type=addsub
  Mult : xbsIndex_r4/Mult  precision=Full  arith_type=Unsigned  n_bits=36  bin_pt=0  quantization=Truncate  overflow=Wrap  en=off  latency=3  use_behavioral_HDL=off  opt=Speed  use_embedded=on  optimum_pipeline=off  pipeline=on  dbl_ovrd=off  use_rpm=on  placement_style=Triangular  block_type=mult
  Mult1 : xbsIndex_r4/Mult  precision=Full  arith_type=Unsigned  n_bits=36  bin_pt=0  quantization=Truncate  overflow=Wrap  en=off  latency=3  use_behavioral_HDL=off  opt=Speed  use_embedded=on  optimum_pipeline=off  pipeline=on  dbl_ovrd=off  use_rpm=on  placement_style=Triangular  block_type=mult
  Reinterpret : xbsIndex_r4/Reinterpret  force_arith_type=on  arith_type="Signed  (2's comp)"  force_bin_pt=on  bin_pt=0  block_type=reinterpret
  Reinterpret1 : xbsIndex_r4/Reinterpret  force_arith_type=on  arith_type="Signed  (2's comp)"  force_bin_pt=on  bin_pt=0  block_type=reinterpret
  Slice_im : xbsIndex_r4/Slice  nbits=20  boolean_output=off  mode=Upper Bit Location + Width  bit1=0  base1=MSB of Input  bit0=0  base0=LSB of Input  dbl_ovrd=off  block_type=slice
  Slice_re : xbsIndex_r4/Slice  nbits=20  boolean_output=off  mode=Upper Bit Location + Width  bit1=0  base1=MSB of Input  bit0=0  base0=LSB of Input  dbl_ovrd=off  block_type=slice
  Out1 : Outport
  wires:
  In2/1 -> Slice_im/1
  In1/1 -> Slice_re/1
  Reinterpret/1 -> Mult/1, Mult/2
  Reinterpret1/1 -> Mult1/2, Mult1/1
  Mult/1 -> AddSub/1
  Mult1/1 -> AddSub/2
  AddSub/1 -> Out1/1
  Slice_re/1 -> Reinterpret/1
  Slice_im/1 -> Reinterpret1/1

== system snap_hdl_pfb_v3/Power_Cal3 ==
  In1 : Inport
  In2 : Inport  Port=2
  AddSub : xbsIndex_r4/AddSub  mode=Addition  use_carryin=off  use_carryout=off  en=off  latency=2  precision=User Defined  arith_type=Unsigned  n_bits=40  bin_pt=0  quantization=Truncate  overflow=Wrap  use_behavioral_HDL=off  hw_selection=Fabric  pipelined=off  dbl_ovrd=off  block_type=addsub
  Mult : xbsIndex_r4/Mult  precision=Full  arith_type=Unsigned  n_bits=36  bin_pt=0  quantization=Truncate  overflow=Wrap  en=off  latency=3  use_behavioral_HDL=off  opt=Speed  use_embedded=on  optimum_pipeline=off  pipeline=on  dbl_ovrd=off  use_rpm=on  placement_style=Triangular  block_type=mult
  Mult1 : xbsIndex_r4/Mult  precision=Full  arith_type=Unsigned  n_bits=36  bin_pt=0  quantization=Truncate  overflow=Wrap  en=off  latency=3  use_behavioral_HDL=off  opt=Speed  use_embedded=on  optimum_pipeline=off  pipeline=on  dbl_ovrd=off  use_rpm=on  placement_style=Triangular  block_type=mult
  Reinterpret : xbsIndex_r4/Reinterpret  force_arith_type=on  arith_type="Signed  (2's comp)"  force_bin_pt=on  bin_pt=0  block_type=reinterpret
  Reinterpret1 : xbsIndex_r4/Reinterpret  force_arith_type=on  arith_type="Signed  (2's comp)"  force_bin_pt=on  bin_pt=0  block_type=reinterpret
  Slice_im : xbsIndex_r4/Slice  nbits=20  boolean_output=off  mode=Upper Bit Location + Width  bit1=0  base1=MSB of Input  bit0=0  base0=LSB of Input  dbl_ovrd=off  block_type=slice
  Slice_re : xbsIndex_r4/Slice  nbits=20  boolean_output=off  mode=Upper Bit Location + Width  bit1=0  base1=MSB of Input  bit0=0  base0=LSB of Input  dbl_ovrd=off  block_type=slice
  Out1 : Outport
  wires:
  In2/1 -> Slice_im/1
  In1/1 -> Slice_re/1
  Reinterpret/1 -> Mult/1, Mult/2
  Reinterpret1/1 -> Mult1/2, Mult1/1
  Mult/1 -> AddSub/1
  Mult1/1 -> AddSub/2
  AddSub/1 -> Out1/1
  Slice_re/1 -> Reinterpret/1
  Slice_im/1 -> Reinterpret1/1

== system snap_hdl_pfb_v3/Sig_sim ==
  Add{,1..3} (4 alike) : Sum
  Band-Limited White Noise{,1..3} (4 alike) : simulink/Sources/Band-Limited White Noise  Cov=[0.01]  Ts=0.1  seed=[23341]
  Sine Wave : Sin  Amplitude=0.2  Frequency=2*3.14*(1/64)  SampleTime=1
  Sine Wave1 : Sin  Amplitude=0.2  Frequency=2*3.14*(1/64)  Phase=2*3.14*(1/128)  SampleTime=1
  Sine Wave2 : Sin  Amplitude=0.2  Frequency=2*3.14*(1/64)  SampleTime=1
  Sine Wave3 : Sin  Amplitude=0.2  Frequency=2*3.14*(1/64)  Phase=2*3.14*(1/128)  SampleTime=1
  Out1 : Outport
  Out2 : Outport  Port=2
  Out3 : Outport  Port=3
  Out4 : Outport  Port=4
  wires:
  Sine Wave/1 -> Add/1
  Sine Wave2/1 -> Add2/1
  Sine Wave3/1 -> Add3/1
  Sine Wave1/1 -> Add1/1
  Band-Limited White Noise/1 -> Add/2
  Add/1 -> Out1/1
  Band-Limited White Noise1/1 -> Add1/2
  Add1/1 -> Out2/1
  Band-Limited White Noise2/1 -> Add2/2
  Add2/1 -> Out3/1
  Band-Limited White Noise3/1 -> Add3/2
  Add3/1 -> Out4/1

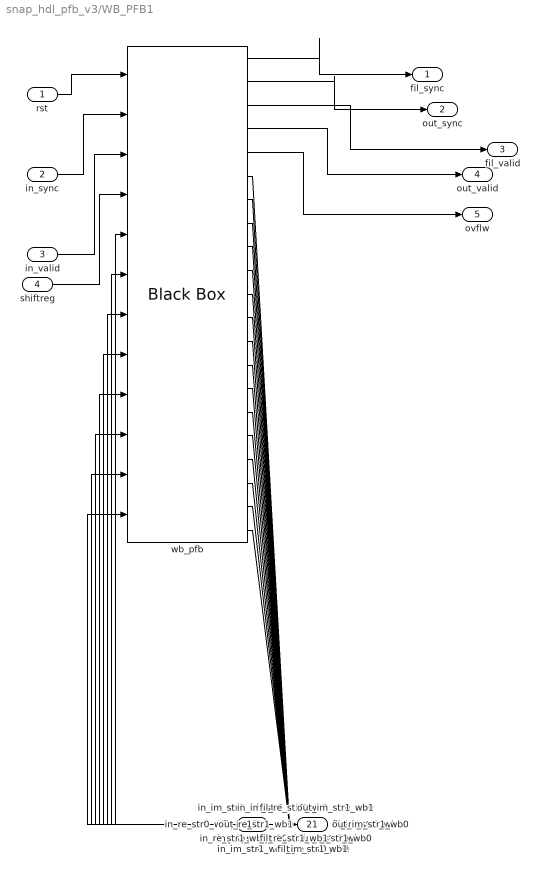
== system snap_hdl_pfb_v3/WB_PFB1 ==
  rst : Inport
  in_sync : Inport  Port=2
  in_valid : Inport  Port=3
  shiftreg : Inport  Port=4
  in_im_str0_wb0 : Inport  Port=5
  in_re_str0_wb0 : Inport  Port=6
  in_im_str0_wb1 : Inport  Port=7
  in_re_str0_wb1 : Inport  Port=8
  in_im_str1_wb0 : Inport  Port=9
  in_re_str1_wb0 : Inport  Port=10
  in_im_str1_wb1 : Inport  Port=11
  in_re_str1_wb1 : Inport  Port=12
  wb_pfb : xbsIndex_r4/Black Box  init_code=wbpfb_unit_top_config  sim_method=ISE Simulator  verbose=off  block_type=blackbox2
  fil_sync : Outport  VectorParamsAs1DForOutWhenUnconnected=off
  out_sync : Outport  Port=2  VectorParamsAs1DForOutWhenUnconnected=off
  fil_valid : Outport  Port=3  VectorParamsAs1DForOutWhenUnconnected=off
  out_valid : Outport  Port=4  VectorParamsAs1DForOutWhenUnconnected=off
  ovflw : Outport  Port=5  VectorParamsAs1DForOutWhenUnconnected=off
  fil_im_str0_wb0 : Outport  Port=6
  fil_re_str0_wb0 : Outport  Port=7
  out_im_str0_wb0 : Outport  Port=8
  out_re_str0_wb0 : Outport  Port=9
  fil_im_str0_wb1 : Outport  Port=10
  fil_re_str0_wb1 : Outport  Port=11
  out_im_str0_wb1 : Outport  Port=12
  out_re_str0_wb1 : Outport  Port=13
  fil_im_str1_wb0 : Outport  Port=14
  fil_re_str1_wb0 : Outport  Port=15
  out_im_str1_wb0 : Outport  Port=16
  out_re_str1_wb0 : Outport  Port=17
  fil_im_str1_wb1 : Outport  Port=18
  fil_re_str1_wb1 : Outport  Port=19
  out_im_str1_wb1 : Outport  Port=20
  out_re_str1_wb1 : Outport  Port=21
  wires:
  rst/1 -> wb_pfb/1
  in_sync/1 -> wb_pfb/2
  in_valid/1 -> wb_pfb/3
  shiftreg/1 -> wb_pfb/4
  wb_pfb/1 -> fil_sync/1
  wb_pfb/2 -> out_sync/1
  wb_pfb/3 -> fil_valid/1
  wb_pfb/4 -> out_valid/1
  wb_pfb/5 -> ovflw/1
  in_im_str0_wb0/1 -> wb_pfb/5
  in_re_str0_wb0/1 -> wb_pfb/6
  wb_pfb/6 -> fil_im_str0_wb0/1
  wb_pfb/7 -> fil_re_str0_wb0/1
  wb_pfb/14 -> out_im_str0_wb0/1
  wb_pfb/15 -> out_re_str0_wb0/1
  in_im_str0_wb1/1 -> wb_pfb/7
  in_re_str0_wb1/1 -> wb_pfb/8
  wb_pfb/8 -> fil_im_str0_wb1/1
  wb_pfb/9 -> fil_re_str0_wb1/1
  wb_pfb/16 -> out_im_str0_wb1/1
  wb_pfb/17 -> out_re_str0_wb1/1
  in_im_str1_wb0/1 -> wb_pfb/9
  in_re_str1_wb0/1 -> wb_pfb/10
  wb_pfb/10 -> fil_im_str1_wb0/1
  wb_pfb/11 -> fil_re_str1_wb0/1
  wb_pfb/18 -> out_im_str1_wb0/1
  wb_pfb/19 -> out_re_str1_wb0/1
  in_im_str1_wb1/1 -> wb_pfb/11
  in_re_str1_wb1/1 -> wb_pfb/12
  wb_pfb/12 -> fil_im_str1_wb1/1
  wb_pfb/13 -> fil_re_str1_wb1/1
  wb_pfb/20 -> out_im_str1_wb1/1
  wb_pfb/21 -> out_re_str1_wb1/1

== system snap_hdl_pfb_v3/acc_len ==
  sim_1 : Inport
  convert1_1 : DataTypeConversion  OutDataTypeStr=fixdt('ufix32_En0')  LockScale=on
  convert2_1 : DataTypeConversion  OutDataTypeStr=fixdt('ufix32_En0')  ConvertRealWorld=Stored Integer (SI)  LockScale=on
  gain_1 : Gain  OutDataTypeStr=fixdt('ufix32_En0')
  io_delay : xbsIndex_r4/Delay  rst=off  infoeditControl=Selection of Reset will increase slice count due to use of real FFs and instead of SRLs  en=off  latency=0  reg_retiming=on  dbl_ovrd=off  block_type=delay
  reint1 : xbsIndex_r4/Reinterpret  force_arith_type=on  arith_type=Unsigned  force_bin_pt=on  bin_pt=0  block_type=reinterpret
  slice_reg : xbsIndex_r4/Slice  nbits=32  boolean_output=off  mode=Lower Bit Location + Width  bit1=0  base1=MSB of Input  bit0=0  base0=LSB of Input  dbl_ovrd=off  block_type=slice
  snap_hdl_pfb_v3_acc_len_user_data_out : xbsIndex_r4/Gateway In  gui_display_data_type=Fixed-point  arith_type=Unsigned  n_bits=32  bin_pt=0  preci_type=Single  exp_width=8  frac_width=24  rows=1  columns=1  quantization="Round  (unbiased: +/- Inf)"  overflow=Saturate  period=1  UseAsADC=off  ADCChannel='1'  interface=None  automatic_assignment=on  address_offset=hex2dec('00')  intf_name=''  intf_description=''  default_value=0  timing_constraint=None  locs_specified=off  LOCs={}  io_standard={}  inherit_from_input=off  hdl_port=on  dbl_ovrd=off  block_type=gatewayin
  in_reg : Outport
  wires:
  snap_hdl_pfb_v3_acc_len_user_data_out/1 -> io_delay/1
  sim_1/1 -> convert1_1/1
  convert1_1/1 -> convert2_1/1
  convert2_1/1 -> gain_1/1
  gain_1/1 -> snap_hdl_pfb_v3_acc_len_user_data_out/1
  io_delay/1 -> slice_reg/1
  slice_reg/1 -> reint1/1
  reint1/1 -> in_reg/1

== system snap_hdl_pfb_v3/led_ctrl ==
  sim_1 : Inport
  convert1_1 : DataTypeConversion  OutDataTypeStr=fixdt('ufix32_En0')  LockScale=on
  convert2_1 : DataTypeConversion  OutDataTypeStr=fixdt('ufix32_En0')  ConvertRealWorld=Stored Integer (SI)  LockScale=on
  gain_1 : Gain  OutDataTypeStr=fixdt('ufix32_En0')
  io_delay : xbsIndex_r4/Delay  rst=off  infoeditControl=Selection of Reset will increase slice count due to use of real FFs and instead of SRLs  en=off  latency=0  reg_retiming=on  dbl_ovrd=off  block_type=delay
  reint1 : xbsIndex_r4/Reinterpret  force_arith_type=on  arith_type=Unsigned  force_bin_pt=on  bin_pt=0  block_type=reinterpret
  slice_reg : xbsIndex_r4/Slice  nbits=32  boolean_output=off  mode=Lower Bit Location + Width  bit1=0  base1=MSB of Input  bit0=0  base0=LSB of Input  dbl_ovrd=off  block_type=slice
  snap_hdl_pfb_v3_led_ctrl_user_data_out : xbsIndex_r4/Gateway In  gui_display_data_type=Fixed-point  arith_type=Unsigned  n_bits=32  bin_pt=0  preci_type=Single  exp_width=8  frac_width=24  rows=1  columns=1  quantization="Round  (unbiased: +/- Inf)"  overflow=Saturate  period=1  UseAsADC=off  ADCChannel='1'  interface=None  automatic_assignment=on  address_offset=hex2dec('00')  intf_name=''  intf_description=''  default_value=0  timing_constraint=None  locs_specified=off  LOCs={}  io_standard={}  inherit_from_input=off  hdl_port=on  dbl_ovrd=off  block_type=gatewayin
  in_reg : Outport
  wires:
  snap_hdl_pfb_v3_led_ctrl_user_data_out/1 -> io_delay/1
  sim_1/1 -> convert1_1/1
  convert1_1/1 -> convert2_1/1
  convert2_1/1 -> gain_1/1
  gain_1/1 -> snap_hdl_pfb_v3_led_ctrl_user_data_out/1
  io_delay/1 -> slice_reg/1
  slice_reg/1 -> reint1/1
  reint1/1 -> in_reg/1

== system snap_hdl_pfb_v3/pfb_status ==
  out_reg : Inport
  assert_reg : xbsIndex_r4/Assert  assert_type=on  type_source=Explicitly  gui_display_data_type=Fixed-point  arith_type=Unsigned  n_bits=12  bin_pt=0  preci_type=Single  exp_width=8  frac_width=24  assert_rate=off  rate_source=Explicitly  period=1  output_port=on  block_type=assert
  cast_gw : xbsIndex_r4/Convert  gui_display_data_type=Fixed-point  arith_type=Unsigned  n_bits=32  bin_pt=0  float_type=Single  exp_bits=8  fraction_bits=24  quantization=Truncate  overflow=Wrap  en=off  latency=1  pipeline=off  dbl_ovrd=off  block_type=convert
  io_delay : xbsIndex_r4/Delay  rst=off  infoeditControl=Selection of Reset will increase slice count due to use of real FFs and instead of SRLs  en=off  latency=0  reg_retiming=on  dbl_ovrd=off  block_type=delay
  reint1 : xbsIndex_r4/Reinterpret  force_arith_type=on  arith_type=Unsigned  force_bin_pt=on  bin_pt=0  block_type=reinterpret
  sim_out : Terminator
  sim_out_reg_gw : xbsIndex_r4/Gateway Out  inherit_from_input=off  hdl_port=off  rows=1  columns=1  UseAsDAC=off  DACChannel='1'  interface=None  automatic_assignment=on  address_offset=hex2dec('00')  intf_name=''  intf_description=''  timing_constraint=None  locs_specified=off  LOCs={}  io_standard={}  block_type=gatewayout
  sim_out_reg_sim_delay : xbsIndex_r4/Delay  rst=off  infoeditControl=Selection of Reset will increase slice count due to use of real FFs and instead of SRLs  en=off  latency=1  reg_retiming=on  dbl_ovrd=off  block_type=delay
  snap_hdl_pfb_v3_pfb_status_user_data_in : xbsIndex_r4/Gateway Out  inherit_from_input=off  hdl_port=on  rows=1  columns=1  UseAsDAC=off  DACChannel='1'  interface=None  automatic_assignment=on  address_offset=hex2dec('00')  intf_name=''  intf_description=''  timing_constraint=None  locs_specified=off  LOCs={}  io_standard={}  block_type=gatewayout
  sim_out_reg : Outport  VectorParamsAs1DForOutWhenUnconnected=off
  wires:
  sim_out_reg_sim_delay/1 -> sim_out_reg_gw/1
  sim_out_reg_gw/1 -> sim_out_reg/1
  io_delay/1 -> cast_gw/1
  cast_gw/1 -> snap_hdl_pfb_v3_pfb_status_user_data_in/1
  snap_hdl_pfb_v3_pfb_status_user_data_in/1 -> sim_out/1
  out_reg/1 -> sim_out_reg_sim_delay/1, assert_reg/1
  assert_reg/1 -> reint1/1
  reint1/1 -> io_delay/1
